simulink model "Tank_Discrete"  (R2024b)
settings: Solver=ode1  StartTime=0.0  StopTime=3600  FixedStep=0.05  RelTol=1e-3
values from neighbouring files (symbols this model uses):
  A1 = 1.5    [init.m]
  A2 = 1.5    [init.m]
  A3 = 1.5    [init.m]
  dt = 0.05    [init.m]
  h1_0 = 0.4    [init.m]
  h2_0 = 0.3    [init.m]
  h3_0 = 0.2    [init.m]
  k_drain = 0.03    [init.m]
undefined symbols (not defined in the file or in its folder): T1, T3
libraries: slpidlib x2
settings Model: Creator=fatjonkabali  LastModifiedBy=fatjonkabali

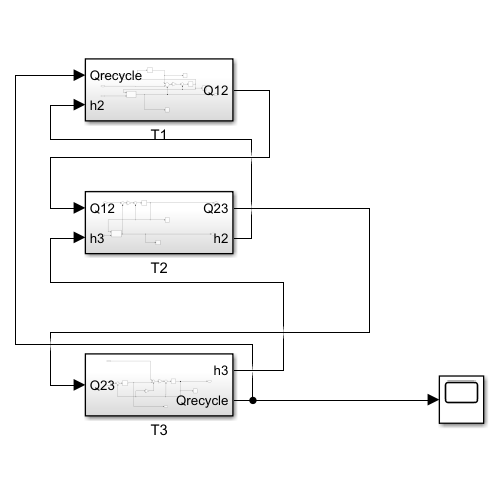
[thumbnail: Simulink's stored preview of the top-level diagram]
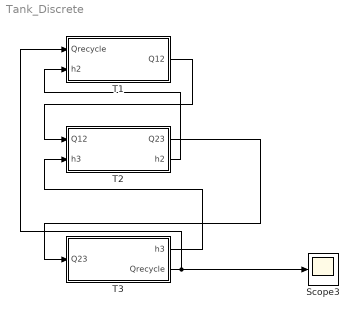
== system Tank_Discrete ==
  Scope3 : Scope
  T1 : Subsystem
  T2 : Subsystem
  T3 : Subsystem
  wires:
  T2/2(h2) -> T1/2(h2)
  T1/1(Q12) -> T2/1(Q12)
  T3/1(h3) -> T2/2(h3)
  T3/2(Qrecycle) -> T1/1(Qrecycle), Scope3/1
  T2/1(Q23) -> T3/1(Q23)

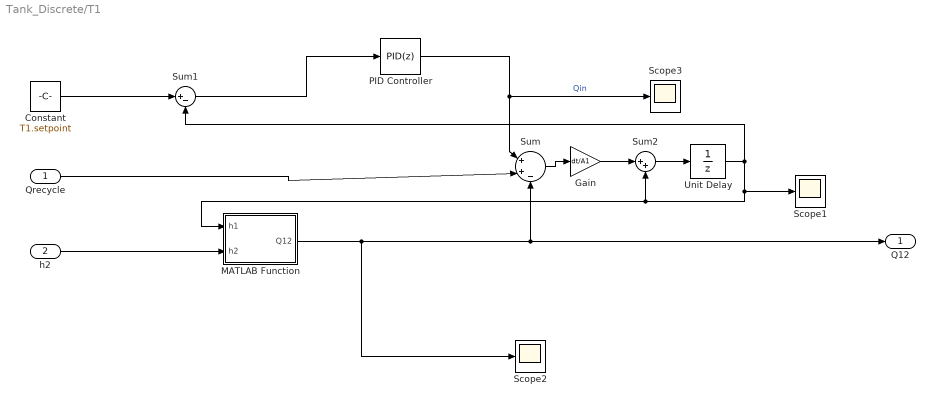
== system Tank_Discrete/T1 ==
  Qrecycle : Inport
  h2 : Inport  Port=2
  Constant : Constant  Value=T1.setpoint
  Gain : Gain  Gain=dt/A1
  MATLAB Function : MATLAB Function  TreatAsAtomicUnit=on
  PID Controller : slpidlib/PID Controller  Controller=PID  Form=Parallel  TimeDomain=Discrete-time  UseExternalTs=off  SampleTime=dt  IntegratorMethod=Forward Euler  FilterMethod=Forward Euler  ControllerParametersSource=internal  P=0.1  I=0.01  UseKiTs=off  D=0.05  UseExternalDerivativeSource=off  N=0  UseFilter=on  TunerSelectOption=Transfer Function Based (PID Tuner App)  InitialConditionSource=internal  InitialConditionForIntegrator=0  InitialConditionForFilter=0  DifferentiatorICPrevScaledInput=0  ExternalReset=none  TrackingMode=off  Kt=1  LimitOutput=on  SatLimitsSource=internal  UpperSaturationLimit=0.5  LowerSaturationLimit=0  LinearizeAsGain=on  AntiWindupMode=none  Kb=1  LimitIntegrator=off  UpperIntegratorSaturationLimit=inf  LowerIntegratorSaturationLimit=-inf  POutMin=[]  POutMax=[]  IOutMin=[]  IOutMax=[]  DOutMin=[]  DOutMax=[]  NOutMin=[]  NOutMax=[]  SumOutMin=[]  SumOutMax=[]  SaturationOutMin=[]  SaturationOutMax=[]  PParamMin=[]  PParamMax=[]  IParamMin=[]  IParamMax=[]  DParamMin=[]  DParamMax=[]  NParamMin=[]  NParamMax=[]  KbParamMin=[]  KbParamMax=[]  KtParamMin=[]  KtParamMax=[]  KbOutMin=[]  KbOutMax=[]  KtOutMin=[]  KtOutMax=[]  IntegratorOutMin=[]  IntegratorOutMax=[]  FilterOutMin=[]  FilterOutMax=[]  SumI1OutMin=[]  SumI1OutMax=[]  SumI2OutMin=[]  SumI2OutMax=[]  SumI3OutMin=[]  SumI3OutMax=[]  SumI4OutMin=[]  SumI4OutMax=[]  SumDOutMin=[]  SumDOutMax=[]  DifferentiatorOutMin=[]  DifferentiatorOutMax=[]  FilterDiffOutCoefMin=[]  FilterDiffOutCoefMax=[]  ReciprocalOutMin=[]  ReciprocalOutMax=[]  SumDenOutMin=[]  SumDenOutMax=[]  SumNumOutMin=[]  SumNumOutMax=[]  DivideOutMin=[]  DivideOutMax=[]  UdiffTsProdOutMin=[]  UdiffTsProdOutMax=[]  NTsProdOutMin=[]  NTsProdOutMax=[]  UintegralTsProdOutMin=[]  UintegralTsProdOutMax=[]  UngainTsProdOutMin=[]  UngainTsProdOutMax=[]  ClampingZeroOutDataTypeStr=Inherit: Inherit via back propagation  ClampingZeroOutMin=[]  ClampingZeroOutMax=[]  FilterDenConstantOutDataTypeStr=Inherit: Inherit via back propagation  FilterDenConstantOutMin=[]  FilterDenConstantOutMax=[]  PCopyOutDataTypeStr=Inherit: Inherit via back propagation  PCopyOutMin=[]  PCopyOutMax=[]  NCopyOutDataTypeStr=Inherit: Inherit via back propagation  NCopyOutMin=[]  NCopyOutMax=[]  IntegratorContinuousStateAttributes=''  IntegratorStateMustResolveToSignalObject=off  IntegratorRTWStateStorageClass=Auto  FilterContinuousStateAttributes=''  FilterStateMustResolveToSignalObject=off  FilterRTWStateStorageClass=Auto  ParallelPVariant=InternalParameters  IdealPVariant=Disabled  IVariant=InternalParameters  DVariant=InternalParameters  IntegratorVariant=Discrete  SatVariant=Enabled  AWVariant=Passthrough  PCopyVariant=Disabled  TRVariant=Disabled  FdbkBlocksVariant=Forward  IdealPFdbkVariant=Disabled  SatFdbkVariant=Disabled  DerivativeFilterVariant=ForwardEulerFilter  NVariant=InternalParameters  NCopyVariant=Disabled  FilterICVariant=InternalICsFilter  IntegratorICVariant=InternalICs  ExternalResetVariant=Disabled  TRSumVariant=Passthrough  SumFdbkVariant=Disabled  SumVariant=Sum_PID  TsampFilterVariant=InternalTs  TsampNgainVariant=Passthrough  TsampIntegralVariant=Disabled_SignalSpec  ExternalSaturationOutDataTypeStr=Inherit: Same as second input  DerivativeSourceVariant=ErrorSignal  PreIntVariant=InternalPreInt
  Scope1 : Scope
  Scope2 : Scope
  Scope3 : Scope
  Sum : Sum  Inputs=|++-
  Sum1 : Sum  Inputs=|+-
  Sum2 : Sum  Inputs=|++
  Unit Delay : UnitDelay  InitialCondition=h1_0  SampleTime=dt  HasFrameUpgradeWarning=on
  Q12 : Outport
  wires:
  MATLAB Function/1(Q12) -> Scope2/1, Q12/1, Sum/3
  Qrecycle/1 -> Sum/2
  PID Controller/1 -> Scope3/1, Sum/1  "Qin"
  Sum/1 -> Gain/1
  Unit Delay/1 -> Sum1/2, Scope1/1, MATLAB Function/1(h1), Sum2/2
  h2/1 -> MATLAB Function/2(h2)
  Sum1/1 -> PID Controller/1
  Constant/1 -> Sum1/1
  Gain/1 -> Sum2/1
  Sum2/1 -> Unit Delay/1

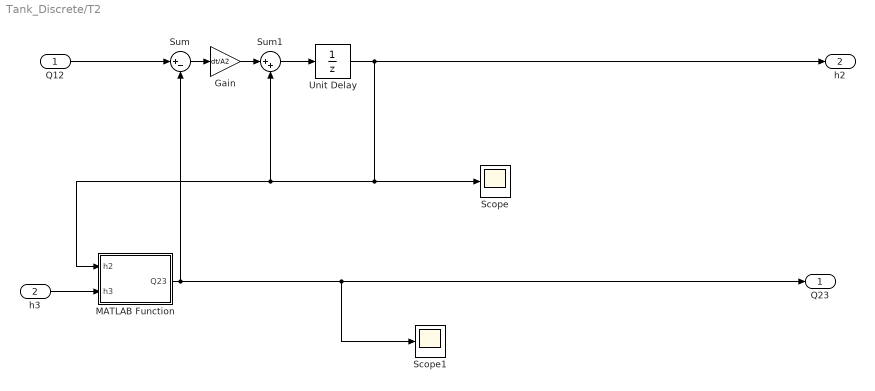
== system Tank_Discrete/T2 ==
  Q12 : Inport
  h3 : Inport  Port=2
  Gain : Gain  Gain=dt/A2
  MATLAB Function : MATLAB Function  TreatAsAtomicUnit=on
  Scope : Scope
  Scope1 : Scope
  Sum : Sum  Inputs=|+-
  Sum1 : Sum  Inputs=|++
  Unit Delay : UnitDelay  InitialCondition=h2_0  SampleTime=dt  HasFrameUpgradeWarning=on
  Q23 : Outport
  h2 : Outport  Port=2
  wires:
  Unit Delay/1 -> Scope/1, Sum1/2, MATLAB Function/1(h2), h2/1
  MATLAB Function/1(Q23) -> Scope1/1, Q23/1, Sum/2
  Q12/1 -> Sum/1
  Sum/1 -> Gain/1
  h3/1 -> MATLAB Function/2(h3)
  Gain/1 -> Sum1/1
  Sum1/1 -> Unit Delay/1

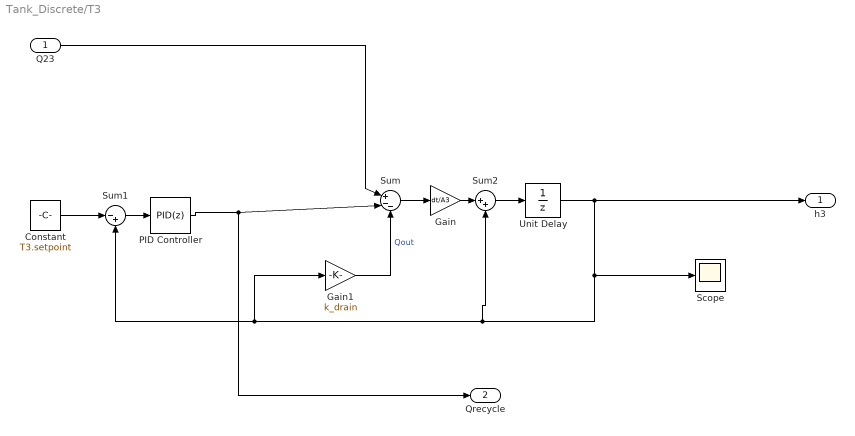
== system Tank_Discrete/T3 ==
  Q23 : Inport
  Constant : Constant  Value=T3.setpoint
  Gain : Gain  Gain=dt/A3
  Gain1 : Gain  Gain=k_drain
  PID Controller : slpidlib/PID Controller  Controller=PID  Form=Parallel  TimeDomain=Discrete-time  UseExternalTs=off  SampleTime=dt  IntegratorMethod=Forward Euler  FilterMethod=Forward Euler  ControllerParametersSource=internal  P=0.1  I=0.01  UseKiTs=off  D=0.05  UseExternalDerivativeSource=off  N=0  UseFilter=on  TunerSelectOption=Transfer Function Based (PID Tuner App)  InitialConditionSource=internal  InitialConditionForIntegrator=0  InitialConditionForFilter=0  DifferentiatorICPrevScaledInput=0  ExternalReset=none  TrackingMode=off  Kt=1  LimitOutput=on  SatLimitsSource=internal  UpperSaturationLimit=0.5  LowerSaturationLimit=0  LinearizeAsGain=on  AntiWindupMode=none  Kb=1  LimitIntegrator=off  UpperIntegratorSaturationLimit=inf  LowerIntegratorSaturationLimit=-inf  POutMin=[]  POutMax=[]  IOutMin=[]  IOutMax=[]  DOutMin=[]  DOutMax=[]  NOutMin=[]  NOutMax=[]  SumOutMin=[]  SumOutMax=[]  SaturationOutMin=[]  SaturationOutMax=[]  PParamMin=[]  PParamMax=[]  IParamMin=[]  IParamMax=[]  DParamMin=[]  DParamMax=[]  NParamMin=[]  NParamMax=[]  KbParamMin=[]  KbParamMax=[]  KtParamMin=[]  KtParamMax=[]  KbOutMin=[]  KbOutMax=[]  KtOutMin=[]  KtOutMax=[]  IntegratorOutMin=[]  IntegratorOutMax=[]  FilterOutMin=[]  FilterOutMax=[]  SumI1OutMin=[]  SumI1OutMax=[]  SumI2OutMin=[]  SumI2OutMax=[]  SumI3OutMin=[]  SumI3OutMax=[]  SumI4OutMin=[]  SumI4OutMax=[]  SumDOutMin=[]  SumDOutMax=[]  DifferentiatorOutMin=[]  DifferentiatorOutMax=[]  FilterDiffOutCoefMin=[]  FilterDiffOutCoefMax=[]  ReciprocalOutMin=[]  ReciprocalOutMax=[]  SumDenOutMin=[]  SumDenOutMax=[]  SumNumOutMin=[]  SumNumOutMax=[]  DivideOutMin=[]  DivideOutMax=[]  UdiffTsProdOutMin=[]  UdiffTsProdOutMax=[]  NTsProdOutMin=[]  NTsProdOutMax=[]  UintegralTsProdOutMin=[]  UintegralTsProdOutMax=[]  UngainTsProdOutMin=[]  UngainTsProdOutMax=[]  ClampingZeroOutDataTypeStr=Inherit: Inherit via back propagation  ClampingZeroOutMin=[]  ClampingZeroOutMax=[]  FilterDenConstantOutDataTypeStr=Inherit: Inherit via back propagation  FilterDenConstantOutMin=[]  FilterDenConstantOutMax=[]  PCopyOutDataTypeStr=Inherit: Inherit via back propagation  PCopyOutMin=[]  PCopyOutMax=[]  NCopyOutDataTypeStr=Inherit: Inherit via back propagation  NCopyOutMin=[]  NCopyOutMax=[]  IntegratorContinuousStateAttributes=''  IntegratorStateMustResolveToSignalObject=off  IntegratorRTWStateStorageClass=Auto  FilterContinuousStateAttributes=''  FilterStateMustResolveToSignalObject=off  FilterRTWStateStorageClass=Auto  ParallelPVariant=InternalParameters  IdealPVariant=Disabled  IVariant=InternalParameters  DVariant=InternalParameters  IntegratorVariant=Discrete  SatVariant=Enabled  AWVariant=Passthrough  PCopyVariant=Disabled  TRVariant=Disabled  FdbkBlocksVariant=Forward  IdealPFdbkVariant=Disabled  SatFdbkVariant=Disabled  DerivativeFilterVariant=ForwardEulerFilter  NVariant=InternalParameters  NCopyVariant=Disabled  FilterICVariant=InternalICsFilter  IntegratorICVariant=InternalICs  ExternalResetVariant=Disabled  TRSumVariant=Passthrough  SumFdbkVariant=Disabled  SumVariant=Sum_PID  TsampFilterVariant=InternalTs  TsampNgainVariant=Passthrough  TsampIntegralVariant=Disabled_SignalSpec  ExternalSaturationOutDataTypeStr=Inherit: Same as second input  DerivativeSourceVariant=ErrorSignal  PreIntVariant=InternalPreInt
  Scope : Scope
  Sum : Sum  Inputs=|+--
  Sum1 : Sum  Inputs=|-+
  Sum2 : Sum  Inputs=|++
  Unit Delay : UnitDelay  InitialCondition=h3_0  SampleTime=dt  HasFrameUpgradeWarning=on
  h3 : Outport
  Qrecycle : Outport  Port=2
  wires:
  Q23/1 -> Sum/1
  Sum/1 -> Gain/1
  Gain1/1 -> Sum/3  "Qout"
  PID Controller/1 -> Qrecycle/1, Sum/2
  Sum1/1 -> PID Controller/1
  Constant/1 -> Sum1/1
  Gain/1 -> Sum2/1
  Sum2/1 -> Unit Delay/1
  Unit Delay/1 -> Scope/1, Sum2/2, Gain1/1, Sum1/2, h3/1

== matlab function Tank_Discrete/T1/MATLAB Function ==
  data: h1 input; Q12 output; h2 input
function Q12 = flow12(h1, h2)
    k1 = 0.8;
    Q12 = k1 * sign(h1 - h2) * sqrt(abs(h1 - h2));
end

== matlab function Tank_Discrete/T2/MATLAB Function ==
  data: h2 input; Q23 output; h3 input
function Q23 = flow23(h2, h3)
    k2 = 0.6;
    Q23 = k2 * sign(h2 - h3) * sqrt(abs(h2 - h3));
end
